simulink model "EE463_SoftwareProject2_q1_SinglePhaseControlledRectifier_a"  (R2018a)
settings: Solver=VariableStepDiscrete  StartTime=0.0  StopTime=0.5  RelTol=1e-3
libraries: powerlib x9
settings Model: Creator=mertelmas  LastModifiedBy=mertelmas

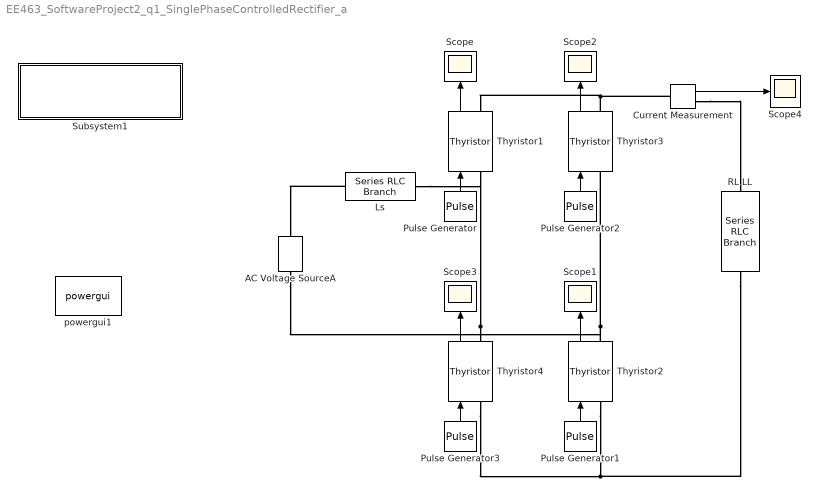
== system EE463_SoftwareProject2_q1_SinglePhaseControlledRectifier_a ==
  AC Voltage SourceA : powerlib/Electrical Sources/AC Voltage Source  Amplitude=326  Phase=0  Frequency=50  SampleTime=0  Measurements=None  BusType=swing  Pref=10e3  Qref=0  Qmin=-inf  Qmax=+inf
  Current Measurement : powerlib/Measurements/Current Measurement  PhasorSimulation=off  OutputType=Complex  PSBequivalent=0
  Ls : powerlib/Elements/Series RLC Branch  LConnTagsString=__new0  RConnTagsString=__new0  BranchType=L  Resistance=1  Inductance=5e-4  SetiL0=off  InitialCurrent=0  Capacitance=1e-6  Setx0=off  InitialVoltage=0  Measurements=None
  Pulse Generator : DiscretePulseGenerator  PulseType=Time based  Period=0.01  PulseWidth=50
  Pulse Generator1 : DiscretePulseGenerator  PulseType=Time based  Period=0.01  PulseWidth=50
  Pulse Generator2 : DiscretePulseGenerator  PulseType=Time based  Period=0.01  PulseWidth=50  PhaseDelay=0.01
  Pulse Generator3 : DiscretePulseGenerator  PulseType=Time based  Period=0.01  PulseWidth=50  PhaseDelay=0.01
  RL LL : powerlib/Elements/Series RLC Branch  LConnTagsString=__new0  RConnTagsString=__new0  BranchType=RL  Resistance=4  Inductance=0.2  SetiL0=off  InitialCurrent=0  Capacitance=1e-6  Setx0=off  InitialVoltage=0  Measurements=None
  Scope{,1..4} (5 alike) : Scope
  Subsystem1 : Subsystem
      settings: OpenFcn=open_system('power_new_palette')
      mask Display: disp(sprintf('Open Simscape Power Systems\n(Specialized Technology)\nPalette Library'));
  Thyristor{1..4} (4 alike) : powerlib/Power Electronics/Thyristor  Ron=0.001  Lon=0  Vf=0.8  IC=0  Rs=500  Cs=250e-9  Measurements=on
  powergui1 : powerlib/powergui  Priority=1  SimulationMode=Discrete  SampleTime=1e-5  frequency=60  Iterations=50  frequencyindice=50  Pbase=100e6  ErrMax=1e-4  UnitsV=kV  UnitsW=MW  buscounter=0  FunctionMessages=off  echomessages=off  EnableUseOfTLC=off  CurrentSourceSwitches=off  DisableSnubberDevices=off  DisableRonSwitches=off  DisableVfSwitches=off  DisplayEquations=off  SolverType=Tustin/Backward Euler (TBE)  Interpol=off  ExternalGateDelay=off  methode=off  Ts=100  x0status=blocks  SPID=off  SwTol=0  HookPort=off  RestoreLinks=warning  ResistiveCurrentMeasurement=off  Frange=[0:2:500]  Ylog=off  Xlog=on  ShowGrid=off  save=off  variable=ZData  structure=0  ZoomFFT=on  StartTime=0.0  cycles=1  DisplayStyle=1  fundamental=60  FreqAxis=off  MaxFrequency=1000  frequencyindicesteady=1  RmsSteady=1  display=off
  wires:
  Thyristor1/1 -> Scope/1
  Pulse Generator/1 -> Thyristor1/1
  Pulse Generator1/1 -> Thyristor2/1
  Thyristor2/1 -> Scope1/1
  Pulse Generator2/1 -> Thyristor3/1
  Thyristor3/1 -> Scope2/1
  Pulse Generator3/1 -> Thyristor4/1
  Thyristor4/1 -> Scope3/1
  Current Measurement/1 -> Scope4/1
  connections:
  Ls/LConn1 -- AC Voltage SourceA/RConn1
  Thyristor4/RConn1 -- Ls/RConn1 -- Thyristor1/LConn1
  AC Voltage SourceA/LConn1 -- Thyristor2/RConn1 -- Thyristor3/LConn1
  Thyristor3/RConn1 -- Current Measurement/LConn1 -- Thyristor1/RConn1
  Thyristor4/LConn1 -- RL LL/RConn1 -- Thyristor2/LConn1
  Current Measurement/RConn1 -- RL LL/LConn1

== system EE463_SoftwareProject2_q1_SinglePhaseControlledRectifier_a/Subsystem1 ==
